simulink model "atrias_2d"  (R2014b)
settings: Solver=ode45  StartTime=0.0  StopTime=t_end
InitFcn:
  | colors
  | simulation_params
  | mechanical_params
StartFcn:
  | tic
StopFcn:
  | stopscript
values from neighbouring files (symbols this model uses):
  A_lpf_velocity = 1 + B1_lpf_velocity + B2_lpf_velocity    [simulation_params.m]
  B1_lpf_velocity = -2*exp(-lpf_damping*fcut_velocity*sample_time)*cos(fcut_velocity*sample_time*sqrt(1-lpf_damping^2))    [simulation_params.m]
  B2_lpf_velocity = exp(-2*lpf_damping*fcut_velocity*sample_time)    [simulation_params.m]
  b_hmotor = 0    [mechanical_params.m]
  b_leg_spring = 0.075*sqrt(k_leg_spring*0.5*.25^2)    [mechanical_params.m]
  b_rotor = 0*60/(2*pi)*9.725e-5    (= 0)    [mechanical_params.m]
  breakaway_friction = [25 25 25 25]    [mechanical_params.m]
  coulomb_friction = [20 20 20 20]    [mechanical_params.m]
  d_com = (d_hip_com_to_torso_com*m_torso)/(m_torso + num_legs*m_hshaft)    [mechanical_params.m]
  delta_phi_max = 160*pi/180    (= 2.79252680319)    [mechanical_params.m]
  delta_phi_min = 25.5*pi/180    (= 0.445058959259)    [mechanical_params.m]
  friction_linear_zone = [0.5 0.5 0.5 0.5].*pi/180    [mechanical_params.m]
  g = 9.81    [mechanical_params.m]
  HIP_MTR_MAX_TORQUE = max_current_hip*Kt_hip*N_h    (= 629.28)    [mechanical_params.m]
  initial_boom_pitch = 0    [mechanical_params.m]
  initial_boom_roll = asin((initial_com_height + boom_mount_to_com + boom_mount_to_center*tan(pitch_mount_angle) - (base_12(2) + yshaft_12(2))) / (l_boom + boom_mount_to_center_diagonal))    [mechanical_params.m]
  initial_boom_yaw = 0    [mechanical_params.m]
  initial_hip_roll = 0*pi/180    (= 0)    [mechanical_params.m]
  initial_winch_angle = -12 * pi/180    (= -0.209439510239)    [mechanical_params.m]
  k_gx = m_total*g/0.01    (= 57082.15332)    [mechanical_params.m]
  k_gy = m_total*g/0.005    (= 114164.30664)    [mechanical_params.m]
  k_leg_spring = 2950    [mechanical_params.m]
  k_phi = 5000    [mechanical_params.m]
  Kb_leg = 0.121    [mechanical_params.m]
  kd_winch = td_winch*kp_winch    (= 989.945961256)    [mechanical_params.m]
  kp_winch = winch_gravity_comp/(3*pi/180)    (= 19798.9192251)    [mechanical_params.m]
  Kt_leg = 0.121    [mechanical_params.m]
  L_leg = 0.102e-3    (= 0.000102)    [mechanical_params.m]
  l_seg = 0.5    [mechanical_params.m]
  LEG_MTR_MAX_TORQUE = max_current_leg * Kt_leg * N    (= 1210)    [mechanical_params.m]
  lowerleg_12 = 0.40    (= 0.4)    [mechanical_params.m]
  m_boom = 4.49    [mechanical_params.m]
  m_fblink = 0.46    [mechanical_params.m]
  m_hshaft = 18    [mechanical_params.m]
  m_lowerleg = 0.4438    [mechanical_params.m]
  m_output_gear = 1e-5    (= 1e-05)    [mechanical_params.m]
  m_rotor = 1e-5    (= 1e-05)    [mechanical_params.m]
  m_shin = 0.75    [mechanical_params.m]
  m_thigh = 0.69    [mechanical_params.m]
  m_torso = 17.5    [mechanical_params.m]
  m_total = num_legs*(m_hshaft + m_thigh + m_lowerleg + m_shin + m_fblink + 2*m_gearing) + m_torso    (= 58.18772)    [mechanical_params.m]
  m_virtual_gear = 1e-5    (= 1e-05)    [mechanical_params.m]
  m_yshaft = 12.89    [mechanical_params.m]
  max_current_leg = 200    [mechanical_params.m]
  max_voltage_leg = 50    [mechanical_params.m]
  mu_hmotor = 0.90    (= 0.9)    [mechanical_params.m]
  mu_motor = 0.85    [mechanical_params.m]
  mu_slide = 0.95    [mechanical_params.m]
  mu_stick = 1.00    (= 1)    [mechanical_params.m]
  N = 50    [mechanical_params.m]
  N_h = r_hip_shaft / r_hip_gearhead    (= 57)    [mechanical_params.m]
  output_sample_time = 1/1000    (= 0.001)    [simulation_params.m]
  phi_max_collision = -5*pi/180    (= -0.0872664625997)    [mechanical_params.m]
  phi_roll_max = pi + 16*pi/180    (= 3.42084533391)    [mechanical_params.m]
  phi_roll_min = pi - 9*pi/180    (= 2.98451302091)    [mechanical_params.m]
  phi_shin_max = 3*pi/2 + 17.5*pi/180    (= 5.01782159948)    [mechanical_params.m]
  phi_shin_min = pi - 45*pi/180    (= 2.35619449019)    [mechanical_params.m]
  phi_thigh_max = pi + 45*pi/180    (= 3.92699081699)    [mechanical_params.m]
  phi_thigh_min = pi/2 - 17.5*pi/180    (= 1.2653637077)    [mechanical_params.m]
  r_hip_gearhead = 0.009525    [mechanical_params.m]
  r_hip_shaft = 0.542925    [mechanical_params.m]
  R_leg = 0.052    [mechanical_params.m]
  r_rotor = 0.001    [mechanical_params.m]
  r_virtual_gear = N*r_rotor    (= 0.05)    [mechanical_params.m]
  s = (x - x1)/(x2 - x1)    [controller.m]
  sample_time = 1/sample_freq    (= 0.001)    [simulation_params.m]
  shin_12 = 0.40    (= 0.4)    [mechanical_params.m]
  shin_initial_l = initial_l_leg_angle + acos(initial_l_leg_length)    [mechanical_params.m]
  shin_initial_r = initial_r_leg_angle + acos(initial_r_leg_length)    [mechanical_params.m]
  thigh_initial_l = initial_l_leg_angle - acos(initial_l_leg_length)    [mechanical_params.m]
  thigh_initial_r = initial_r_leg_angle - acos(initial_r_leg_length)    [mechanical_params.m]
  tile_color = cmap(floor((tile_scale/(max_floor_tile_height+eps))*length(cmap))+1,:)    [mechanical_params.m]
  tile_cross_section = [1.5 0.03; 1.5 0; 3 0; 3 0.03]    [mechanical_params.m]
  tile_delta = [0 1; 0 0; 0 0; 0 1]    [mechanical_params.m]
  tile_scale = zeros(12, 1)    [mechanical_params.m]
  v_gx_max = 0.03    [mechanical_params.m]
  v_gy_max = 0.03    [mechanical_params.m]
  v_phi_max = 1/60    (= 0.0166666666667)    [mechanical_params.m]
  viscous_friction = [0.001 0.001 0.001 0.001]    [mechanical_params.m]
  vLimit = 0.01    [mechanical_params.m]
undefined symbols (not defined in the file or in its folder): base_color_d, boom_color_d, fblink_color_d, floor_color_d, hshaft_color_d, lowerleg_color_d, rad, sgn, shin_color_d, t_friction, thigh_color_d, torso_color_d, X, Y, yshaft_color_d, Z
libraries: sm_lib x196, nesl_utility x125, simulink x48, fl_lib x16, simulink_extras x2, mblibv1 x2, commnoisgen2 x1
(part 5 of 8)

== system atrias_2d/Mechanical Simulation Layer/R Leg/Shin SEA ==
  note: Shin SEA Mechanics
  Shin Gear Torque [Nm] : Inport
  Shin Joint [rad rad/s] : Inport  Port=2
  Demux : Demux  Outputs=2
  Gain : Gain  Gain=k_leg_spring
  Gain1 : Gain  Gain=b_leg_spring
  Initial Gear Angle : Constant  Value=shin_initial_r
  Inverse Gear Ratio2 : Gain  Gain=1/N
  Inverse Gear Ratio3 : Gain  Gain=Kt_leg
  Inverse Gear Ratio4 : Gain  Gain=1/Kt_leg
  Motor Efficiency : Gain  Gain=mu_motor
  Motor Controller : Subsystem  Commented=on
  Motor Electromagnetism : Subsystem  Commented=on
  Rotor Damping : Gain  Gain=b_rotor
  Rotor and Gearing : Subsystem
  Sum : Sum  Inputs=++|
  Sum2 : Sum  Inputs=+|-
  Sum3 : Sum  Inputs=|+-
  Sum4 : Sum  Inputs=+|-
  Sum5 : Sum  Inputs=|++
  Torque Limiter (outside) 2 : Saturate  UpperLimit=LEG_MTR_MAX_TORQUE  LowerLimit=-LEG_MTR_MAX_TORQUE  ZeroCross=off
      settings: AttributesFormatString=Hi: %<UpperLimit>\nLo: %<LowerLimit>
  Rotor Joint Conn : PMIOPort  Port=1  Side=Left
  Shin Joint Torque [Nm] : Outport
  Shin Gear [rad] : Outport  Port=2
  wires:
  Sum2/1 -> Gain/1
  Sum5/1 -> Rotor and Gearing/2(Spring Torque [Nm]), Shin Joint Torque [Nm]/1
  Sum3/1 -> Motor Efficiency/1
  Rotor Damping/1 -> Sum3/2
  Gain/1 -> Sum5/1  "tau_load"
  Gain1/1 -> Sum5/2
  Sum4/1 -> Gain1/1
  Shin Joint [rad rad/s]/1 -> Demux/1
  Demux/1 -> Sum2/2
  Demux/2 -> Sum4/2
  Inverse Gear Ratio3/1 -> Sum3/1
  Initial Gear Angle/1 -> Sum/1
  Sum/1 -> Shin Gear [rad]/1, Sum2/1
  Rotor and Gearing/1(Gearhead Position [rad]) -> Sum/2
  Rotor and Gearing/2(Gearhead Velocity [rad/s]) -> Sum4/1
  Motor Efficiency/1 -> Rotor and Gearing/1(Rotor Torque [Nm])
  Inverse Gear Ratio4/1 -> Inverse Gear Ratio3/1
  Motor Controller/1(Voltage [V]) -> Motor Electromagnetism/1(Voltage [V])
  Motor Electromagnetism/1(Current [A]) -> Motor Controller/2(Measured Current [A])
  Shin Gear Torque [Nm]/1 -> Torque Limiter (outside) 2/1
  Inverse Gear Ratio2/1 -> Inverse Gear Ratio4/1
  Rotor and Gearing/3(Rotor Velocity [rad/s]) -> Rotor Damping/1
  Torque Limiter (outside) 2/1 -> Inverse Gear Ratio2/1
  connections:
  Rotor and Gearing/LConn1 -- Rotor Joint Conn/RConn1

== system atrias_2d/Mechanical Simulation Layer/R Leg/Thigh ==
  CS1 to CS2 : sm_lib/Frames and Transforms/Rigid Transform  TranslationMethod=Cartesian  TranslationLengthUnit=m  TranslationStandardAxis=+Z  TranslationStandardOffset=0  TranslationCartesianOffset=[0 -l_seg 0]  TranslationROffset=0  TranslationROffsetUnits=m  TranslationZOffset=0  TranslationZOffsetUnits=m  TranslationThetaOffset=0  TranslationThetaOffsetUnits=deg  RotationMethod=None  RotationAngleUnits=deg  RotationStandardAxis=+Z  RotationAngle=0  RotationArbitraryAxis=[0 0 1]  FollAlignAxisA=+X  BaseAlignAxisA=+Y  FollAlignAxisB=+Y  BaseAlignAxisB=+Z  RotationMatrix=[1 0 0; 0 1 0; 0 0 1]  BlockFunction=simmechanics.library.frames_transforms.rigid_transform
  Frame Data : Subsystem
  Solid : sm_lib/Body Elements/Solid  InertiaType=Custom  Mass=m_thigh  MassUnits=kg  CenterOfMass=com_thigh  CenterOfMassUnits=m  MomentsOfInertia=i_thigh_moments  MomentsOfInertiaUnits=kg*m^2  ProductsOfInertia=i_thigh_products  ProductsOfInertiaUnits=kg*m^2  DensityBased=on  Density=1000  DensityUnits=kg/(m^3)  GraphicType=FromGeometry  MarkerShape=Sphere  MarkerSize=10  MarkerSizeUnits=m  GraphicVisPropType=AdvancedVisualProperties  GraphicDiffuseColor=thigh_color_d  GraphicSpecularColor=[0.5 0.5 0.5 1.0]  GraphicAmbientColor=[thigh_color_d*0.5 1.0]  GraphicEmissiveColor=[0.0 0.0 0.0 1.0]  GraphicShininess=128  GraphicOpacity=1.0  GeometryShape=FromFile  RectangleSize=[1 1]  RectangleSizeUnits=m  BrickDimensions=[1 1 1]  BrickDimensionUnits=m  CylinderRadius=l_rad  CylinderRadiusUnits=m  CylinderLength=l_seg  CylinderLengthUnits=m  SphereRadius=1  SphereRadiusUnits=m  EllipsoidRadii=[1 1 1]  EllipsoidRadiiUnits=m  ExtrusionCrossSection=[1 1; -1 1; -1 -1; 1 -1]  ExtrusionCrossSectionUnits=m  ExtrusionLength=1  ExtrusionLengthUnits=m  PolygonNumSides=3  PolygonOuterRadius=1  PolygonOuterRadiusUnits=m  ExtGeomFileType=STL  ExtGeomFileName=thigh.stl  ExtGeomFileUnits=m  RevolutionCrossSection=[1 1; 1 -1; 2 -1; 2 1]  RevolutionCrossSectionUnits=m  RevolutionExtent=Full  RevolutionAngle=180  RevolutionAngleUnits=deg  BlockFunction=simmechanics.library.body_elements.solid
  CS1 : PMIOPort  Port=1  Side=Left
  CS2 : PMIOPort  Port=2  Side=Right
  connections:
  CS2/RConn1 -- CS1 to CS2/RConn1
  CS1 to CS2/LConn1 -- Solid/RConn1 -- Frame Data/LConn1 -- CS1/RConn1

== system atrias_2d/Mechanical Simulation Layer/R Leg/Thigh SEA ==
  note: Thigh SEA Mechanics
  Thigh Gear Torque [Nm] : Inport
  Thigh Joint [rad rad/s] : Inport  Port=2
  Continuous Angle : mblibv1/Utilities/Continuous Angle  rad=rad  rads=rad/s
  Demux : Demux  Outputs=2
  Gain : Gain  Gain=k_leg_spring
  Gain1 : Gain  Gain=b_leg_spring
  Initial Gear Angle : Constant  Value=thigh_initial_r
  Inverse Gear Ratio1 : Gain  Gain=1/N
  Inverse Gear Ratio2 : Gain  Gain=Kt_leg
  Inverse Gear Ratio3 : Gain  Gain=1/Kt_leg
  Motor Efficiency : Gain  Gain=mu_motor
  Motor Controller : Subsystem  Commented=on
  Motor Electromagnetism : Subsystem  Commented=on
  Rotor Damping : Gain  Gain=b_rotor
  Rotor and Gearing : Subsystem
  Sum : Sum  Inputs=++|
  Sum2 : Sum  Inputs=+|-
  Sum3 : Sum  Inputs=|+-
  Sum4 : Sum  Inputs=+|-
  Sum5 : Sum  Inputs=|++
  Torque Limiter (outside) 2 : Saturate  UpperLimit=LEG_MTR_MAX_TORQUE  LowerLimit=-LEG_MTR_MAX_TORQUE  ZeroCross=off
      settings: AttributesFormatString=Hi: %<UpperLimit>\nLo: %<LowerLimit>
  Rotor Joint Conn : PMIOPort  Port=1  Side=Left
  Thigh Joint Torque [Nm] : Outport
  Thigh Gear [rad] : Outport  Port=2
  wires:
  Sum2/1 -> Gain/1
  Sum3/1 -> Motor Efficiency/1
  Rotor Damping/1 -> Sum3/2
  Gain/1 -> Sum5/1  "tau_load"
  Gain1/1 -> Sum5/2
  Sum4/1 -> Gain1/1
  Thigh Joint [rad rad/s]/1 -> Demux/1
  Demux/1 -> Sum2/2
  Demux/2 -> Sum4/2
  Inverse Gear Ratio3/1 -> Inverse Gear Ratio2/1
  Inverse Gear Ratio2/1 -> Sum3/1
  Initial Gear Angle/1 -> Sum/1
  Sum/1 -> Thigh Gear [rad]/1, Sum2/1
  Continuous Angle/1 -> Sum/2
  Rotor and Gearing/1(Gearhead Position [rad]) -> Continuous Angle/1
  Motor Controller/1(Voltage [V]) -> Motor Electromagnetism/1(Voltage [V])
  Motor Electromagnetism/1(Current [A]) -> Motor Controller/2(Measured Current [A])
  Thigh Gear Torque [Nm]/1 -> Torque Limiter (outside) 2/1
  Inverse Gear Ratio1/1 -> Inverse Gear Ratio3/1
  Motor Efficiency/1 -> Rotor and Gearing/1(Rotor Torque [Nm])
  Rotor and Gearing/2(Gearhead Velocity [rad/s]) -> Sum4/1, Continuous Angle/2
  Sum5/1 -> Thigh Joint Torque [Nm]/1, Rotor and Gearing/2(Spring Torque [Nm])
  Rotor and Gearing/3(Rotor Velocity [rad/s]) -> Rotor Damping/1
  Torque Limiter (outside) 2/1 -> Inverse Gear Ratio1/1
  connections:
  Rotor and Gearing/LConn1 -- Rotor Joint Conn/RConn1

== system atrias_2d/Mechanical Simulation Layer/Right Hip Roll Joint/Mechanical Limits  ==
  vphi : Inport
  phi : Inport  Port=2
  Compare To Constant5 : simulink/Logic and Bit Operations/Compare To Constant  relop=<=  const=phi_max_collision  OutDataTypeStr=boolean  ZeroCross=off
  Compare To Zero1 : simulink/Logic and Bit Operations/Compare To Zero  relop=<=  OutDataTypeStr=boolean  ZeroCross=off
  Compare To Zero2 : simulink/Logic and Bit Operations/Compare To Zero  relop=<=  OutDataTypeStr=boolean  ZeroCross=off
  Constant1 : Constant  Value=phi_roll_min
  Constant2 : Constant  Value=phi_roll_max
  Enabled Subsystem : Subsystem  TreatAsAtomicUnit=on
  Gain2 : Gain  Gain=-1
  Logical Operator : Logic  Operator=OR  Inputs=1  AllPortsSameDT=off  OutDataTypeStr=boolean
  Mux : Mux  Inputs=2
  Roll Max Collision Model : Subsystem
  Roll Min Collision Model : Subsystem
  Stop Simulation6 : Stop
  Sum1 : Sum  Inputs=-+|
  Sum11 : Sum  Inputs=-|+
  Sum5 : Sum  Inputs=+-|
  tau_reaction : Outport
  wires:
  Sum1/1 -> [col_hip_min], Compare To Zero1/1, Roll Min Collision Model/1(phi [rad])
  Roll Min Collision Model/1(tau_interaction[Nm]) -> Sum11/2
  Compare To Zero1/1 -> Roll Min Collision Model/Enable
  phi/1 -> Sum1/2, Sum5/2
  Logical Operator/1 -> Stop Simulation6/1, Enabled Subsystem/Enable
  [col_hip_max] -> Mux/1
  Mux/1 -> Compare To Constant5/1
  [col_hip_min] -> Mux/2
  Sum11/1 -> tau_reaction/1
  Constant1/1 -> Sum1/1
  Compare To Constant5/1 -> Enabled Subsystem/1(Col_Flags), Logical Operator/1
  Constant2/1 -> Sum5/1
  Sum5/1 -> [col_hip_max], Compare To Zero2/1, Roll Max Collision Model/1(phi [rad])
  Compare To Zero2/1 -> Roll Max Collision Model/Enable
  Roll Max Collision Model/1(tau_interaction[Nm]) -> Sum11/1
  vphi/1 -> Roll Min Collision Model/2(vphi [rad/s]), Gain2/1
  Gain2/1 -> Roll Max Collision Model/2(vphi [rad/s])

== system atrias_2d/Mechanical Simulation Layer/Torso/COM Sensor ==
  Mux : Mux  Inputs=3
  PS-Simulink Converter{1,3..8} (7 alike) : nesl_utility/PS-Simulink Converter  PhysicalDomain=network_engine_domain  SubClassName=ps_output  LeftPortType=input  RightPortType=output  PseudoPeriodic=off  Frequencies=[]  Unit=1  AffineConversion=off
  Transform Sensor : sm_lib/Frames and Transforms/Transform Sensor  MeasurementFrame=World  SenseAngle=off  SenseAxis=off  SenseAngle1=off  SenseAngle2=off  SenseAngle3=off  SenseQ=off  SenseR=off  SenseOmegaX=off  SenseOmegaY=off  SenseOmegaZ=off  SenseOmega1=off  SenseOmega2=off  SenseOmega3=off  SenseQDot=off  SenseRDot=off  SenseAlphaX=off  SenseAlphaY=off  SenseAlphaZ=off  SenseAlpha1=off  SenseAlpha2=off  SenseAlpha3=off  SenseQDDot=off  SenseRDDot=off  SenseX=off  SenseY=on  SenseZ=off  SenseRad=off  SenseAzim=off  SenseDist=off  SenseInc=off  SenseXDot=on  SenseYDot=on  SenseZDot=on  SenseRadDot=off  SenseAzimDot=off  SenseDistDot=off  SenseIncDot=off  SenseXDDot=on  SenseYDDot=on  SenseZDDot=on  SenseRadDDot=off  SenseAzimDDot=off  SenseDistDDot=off  SenseIncDDot=off  BlockFunction=simmechanics.library.frames_transforms.transform_sensor
  Transverse Component : Subsystem
  World Frame : sm_lib/Frames and Transforms/World Frame  BlockFunction=simmechanics.library.frames_transforms.world_frame
  COM : PMIOPort  Port=1  Side=Left
  Acceleration : Outport
  y : Outport  Port=2
  dx : Outport  Port=3
  dy : Outport  Port=4
  wires:
  PS-Simulink Converter5/1 -> Mux/3
  Mux/1 -> Acceleration/1
  PS-Simulink Converter8/1 -> y/1
  PS-Simulink Converter3/1 -> Mux/2
  PS-Simulink Converter4/1 -> Mux/1
  PS-Simulink Converter7/1 -> Transverse Component/1(x)
  Transverse Component/1(transverse) -> dx/1
  [qYaw] -> Transverse Component/3(yaw)
  PS-Simulink Converter1/1 -> dy/1
  PS-Simulink Converter6/1 -> Transverse Component/2(z)
  connections:
  COM/RConn1 -- Transform Sensor/RConn1
  World Frame/RConn1 -- Transform Sensor/LConn1
  PS-Simulink Converter5/LConn1 -- Transform Sensor/RConn8
  PS-Simulink Converter3/LConn1 -- Transform Sensor/RConn7
  PS-Simulink Converter4/LConn1 -- Transform Sensor/RConn6
  PS-Simulink Converter6/LConn1 -- Transform Sensor/RConn5
  PS-Simulink Converter7/LConn1 -- Transform Sensor/RConn3
  PS-Simulink Converter8/LConn1 -- Transform Sensor/RConn2
  PS-Simulink Converter1/LConn1 -- Transform Sensor/RConn4

== system atrias_2d/Mechanical Simulation Layer/Torso/Frame Data ==
  Kinematic Data : ToWorkspace  VariableName=torso_out  SampleTime=output_sample_time
      settings: Save2DSignal=2-D array (concatenate along first dimension)
  Mux : Mux
  PS-Simulink Converter{,1..3} (4 alike) : nesl_utility/PS-Simulink Converter  PhysicalDomain=network_engine_domain  SubClassName=ps_output  LeftPortType=input  RightPortType=output  PseudoPeriodic=off  Frequencies=[]  Unit=1  AffineConversion=off
  Transform Sensor : sm_lib/Frames and Transforms/Transform Sensor  MeasurementFrame=World  SenseAngle=off  SenseAxis=off  SenseAngle1=off  SenseAngle2=off  SenseAngle3=off  SenseQ=on  SenseR=off  SenseOmegaX=off  SenseOmegaY=off  SenseOmegaZ=off  SenseOmega1=off  SenseOmega2=off  SenseOmega3=off  SenseQDot=off  SenseRDot=off  SenseAlphaX=off  SenseAlphaY=off  SenseAlphaZ=off  SenseAlpha1=off  SenseAlpha2=off  SenseAlpha3=off  SenseQDDot=off  SenseRDDot=off  SenseX=on  SenseY=on  SenseZ=on  SenseRad=off  SenseAzim=off  SenseDist=off  SenseInc=off  SenseXDot=off  SenseYDot=off  SenseZDot=off  SenseRadDot=off  SenseAzimDot=off  SenseDistDot=off  SenseIncDot=off  SenseXDDot=off  SenseYDDot=off  SenseZDDot=off  SenseRadDDot=off  SenseAzimDDot=off  SenseDistDDot=off  SenseIncDDot=off  BlockFunction=simmechanics.library.frames_transforms.transform_sensor
  World Frame : sm_lib/Frames and Transforms/World Frame  BlockFunction=simmechanics.library.frames_transforms.world_frame
  Frame : PMIOPort  Port=1  Side=Left
  wires:
  Mux/1 -> Kinematic Data/1
  PS-Simulink Converter/1 -> Mux/1
  PS-Simulink Converter1/1 -> Mux/2
  PS-Simulink Converter2/1 -> Mux/3
  PS-Simulink Converter3/1 -> Mux/4
  connections:
  PS-Simulink Converter3/LConn1 -- Transform Sensor/RConn5
  PS-Simulink Converter2/LConn1 -- Transform Sensor/RConn4
  PS-Simulink Converter1/LConn1 -- Transform Sensor/RConn3
  PS-Simulink Converter/LConn1 -- Transform Sensor/RConn2
  Transform Sensor/RConn1 -- Frame/RConn1
  Transform Sensor/LConn1 -- World Frame/RConn1

== system atrias_2d/Mechanical Simulation Layer/Yaw Shaft/Frame Data ==
  Kinematic Data : ToWorkspace  VariableName=boom_yaw_out  SampleTime=output_sample_time
      settings: Save2DSignal=2-D array (concatenate along first dimension)
  Mux : Mux
  PS-Simulink Converter{,1..3} (4 alike) : nesl_utility/PS-Simulink Converter  PhysicalDomain=network_engine_domain  SubClassName=ps_output  LeftPortType=input  RightPortType=output  PseudoPeriodic=off  Frequencies=[]  Unit=1  AffineConversion=off
  Transform Sensor : sm_lib/Frames and Transforms/Transform Sensor  MeasurementFrame=World  SenseAngle=off  SenseAxis=off  SenseAngle1=off  SenseAngle2=off  SenseAngle3=off  SenseQ=on  SenseR=off  SenseOmegaX=off  SenseOmegaY=off  SenseOmegaZ=off  SenseOmega1=off  SenseOmega2=off  SenseOmega3=off  SenseQDot=off  SenseRDot=off  SenseAlphaX=off  SenseAlphaY=off  SenseAlphaZ=off  SenseAlpha1=off  SenseAlpha2=off  SenseAlpha3=off  SenseQDDot=off  SenseRDDot=off  SenseX=on  SenseY=on  SenseZ=on  SenseRad=off  SenseAzim=off  SenseDist=off  SenseInc=off  SenseXDot=off  SenseYDot=off  SenseZDot=off  SenseRadDot=off  SenseAzimDot=off  SenseDistDot=off  SenseIncDot=off  SenseXDDot=off  SenseYDDot=off  SenseZDDot=off  SenseRadDDot=off  SenseAzimDDot=off  SenseDistDDot=off  SenseIncDDot=off  BlockFunction=simmechanics.library.frames_transforms.transform_sensor
  World Frame : sm_lib/Frames and Transforms/World Frame  BlockFunction=simmechanics.library.frames_transforms.world_frame
  Frame : PMIOPort  Port=1  Side=Left
  wires:
  Mux/1 -> Kinematic Data/1
  PS-Simulink Converter/1 -> Mux/1
  PS-Simulink Converter1/1 -> Mux/2
  PS-Simulink Converter2/1 -> Mux/3
  PS-Simulink Converter3/1 -> Mux/4
  connections:
  PS-Simulink Converter3/LConn1 -- Transform Sensor/RConn5
  PS-Simulink Converter2/LConn1 -- Transform Sensor/RConn4
  PS-Simulink Converter1/LConn1 -- Transform Sensor/RConn3
  PS-Simulink Converter/LConn1 -- Transform Sensor/RConn2
  Transform Sensor/RConn1 -- Frame/RConn1
  Transform Sensor/LConn1 -- World Frame/RConn1

== system atrias_2d/Mechanical Simulation Layer/L Ground Contact/Ground Friction Model/Friction Switch ==
  note: Static/Kinetic Friction Switch
  Slide! : Inport
  Stick! : Inport  Port=2
  Memory : Memory  InheritSampleTime=on
  S-R Flip-Flop : simulink_extras/Flip Flops/S-R Flip-Flop  initial_condition=0
  Terminator : Terminator
  Stiction : Outport
  wires:
  S-R Flip-Flop/1 -> Memory/1
  S-R Flip-Flop/2 -> Terminator/1
  Stick!/1 -> S-R Flip-Flop/1
  Slide!/1 -> S-R Flip-Flop/2
  Memory/1 -> Stiction/1

== system atrias_2d/Mechanical Simulation Layer/L Ground Contact/Ground Friction Model/t-Axis Kinetic Friction Model ==
  note: Kinetic Friction Model
  note: Footpoint Determiner
  note: Sliding Limit Detector
  pos_x [m] : Inport
  vel_x [m/s] : Inport  Port=2
  pos_z [m] : Inport  Port=3
  vel_z [m/s] : Inport  Port=4
  F_Normal [N] : Inport  Port=5
  Enable : EnablePort  StatesWhenEnabling=reset  ZeroCross=off
  Constant : Constant  Value=vLimit
  Constant1 : Constant  Value=eps
  Demux : Demux  Outputs=2
  Divide : Product  Inputs=*/
  FixPt Relational Operator : RelationalOperator  Operator=>  OutDataTypeStr=boolean  ZeroCross=off
  Magnitude : Subsystem
  Memory : Memory  InheritSampleTime=on
  Mux : Mux  Inputs=2
  Negative : simulink/Logic and Bit Operations/Compare To Zero  relop=<  OutDataTypeStr=boolean
  Product : Product  RndMeth=Zero
  Sum : Sum  Inputs=|+-
  Sum1 : Sum  Inputs=|++
  reverse : Gain  Gain=-1
  sliding friction coefficient : Gain  Gain=mu_slide
  posFP_x [m] : Outport  InitialOutput=0
      settings: AttributesFormatString=initial = '%<InitialOutput>'\nwhen disabled = '%<OutputWhenDisabled>'
  posFP_z [m] : Outport  Port=2  InitialOutput=0
      settings: AttributesFormatString=initial = '%<InitialOutput>'\nwhen disabled = '%<OutputWhenDisabled>'
  Stiction! : Outport  Port=3  OutputWhenDisabled=reset  InitialOutput=0
      settings: AttributesFormatString=initial = '%<InitialOutput>'\nwhen disabled = '%<OutputWhenDisabled>'
  Fx_Slide [N] : Outport  Port=4  OutputWhenDisabled=reset  InitialOutput=0
      settings: AttributesFormatString=initial = '%<InitialOutput>'\nwhen disabled = '%<OutputWhenDisabled>'
  Fz_Slide [N] : Outport  Port=5  OutputWhenDisabled=reset  InitialOutput=0
      settings: AttributesFormatString=initial = '%<InitialOutput>'\nwhen disabled = '%<OutputWhenDisabled>'
  wires:
  reverse/1 -> Product/1
  F_Normal [N]/1 -> sliding friction coefficient/1
  pos_x [m]/1 -> posFP_x [m]/1
  sliding friction coefficient/1 -> Product/2
  Divide/1 -> reverse/1
  FixPt Relational Operator/1 -> Stiction!/1
  Memory/1 -> FixPt Relational Operator/2
  Negative/1 -> Memory/1, FixPt Relational Operator/1
  Magnitude/1(Magnitude) -> Sum/1, Sum1/1
  Sum/1 -> Negative/1
  Constant/1 -> Sum/2
  pos_z [m]/1 -> posFP_z [m]/1
  vel_x [m/s]/1 -> Mux/1
  vel_z [m/s]/1 -> Mux/2
  Mux/1 -> Divide/1, Magnitude/1(Vector)
  Constant1/1 -> Sum1/2
  Sum1/1 -> Divide/2
  Product/1 -> Demux/1
  Demux/1 -> Fx_Slide [N]/1
  Demux/2 -> Fz_Slide [N]/1

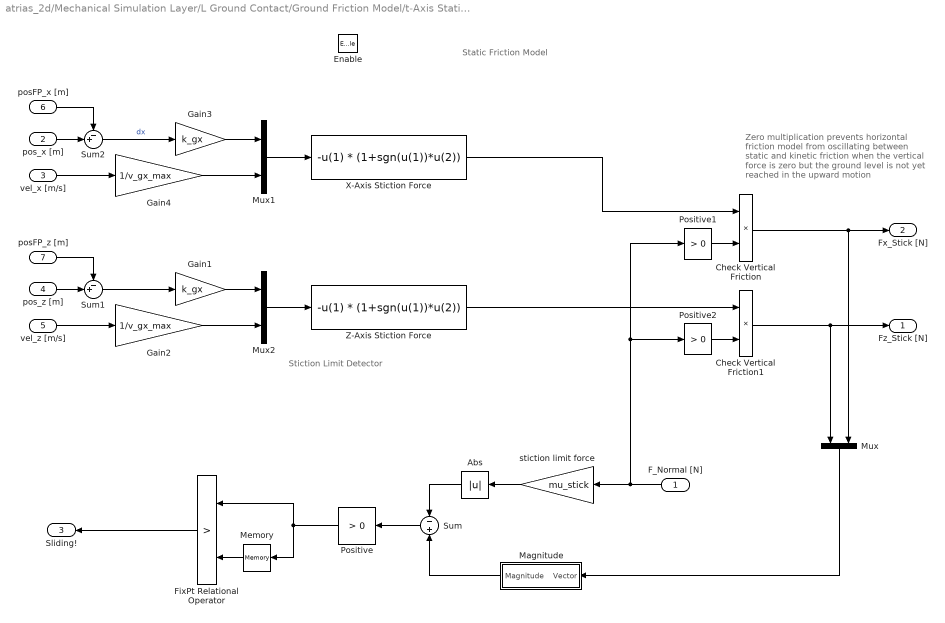
== system atrias_2d/Mechanical Simulation Layer/L Ground Contact/Ground Friction Model/t-Axis Static Friction Model ==
  note: Zero multiplication prevents
      | horizontal friction model from
      | oscillating between static and kinetic
      | friction when the vertical force is zero but
      | the ground level is not yet reached
      | in the upward motion
  note: Stiction Limit Detector
  note: Static Friction Model
  F_Normal [N] : Inport
  pos_x [m] : Inport  Port=2
  vel_x [m/s] : Inport  Port=3
  pos_z [m] : Inport  Port=4
  vel_z [m/s] : Inport  Port=5
  posFP_x [m] : Inport  Port=6
  posFP_z [m] : Inport  Port=7
  Enable : EnablePort  StatesWhenEnabling=reset  ZeroCross=off
  Abs : Abs
  Check Vertical Friction : Product  RndMeth=Zero
  Check Vertical Friction1 : Product  RndMeth=Zero
  FixPt Relational Operator : RelationalOperator  Operator=>  OutDataTypeStr=boolean  ZeroCross=off
  Gain1 : Gain  Gain=k_gx
  Gain2 : Gain  Gain=1/v_gx_max
  Gain3 : Gain  Gain=k_gx
  Gain4 : Gain  Gain=1/v_gx_max
  Magnitude : Subsystem
  Memory : Memory  InheritSampleTime=on
  Mux : Mux  Inputs=2
  Mux1 : Mux  Inputs=2
  Mux2 : Mux  Inputs=2
  Positive : simulink/Logic and Bit Operations/Compare To Zero  relop=>  OutDataTypeStr=boolean
  Positive1 : simulink/Logic and Bit Operations/Compare To Zero  relop=>  OutDataTypeStr=boolean
  Positive2 : simulink/Logic and Bit Operations/Compare To Zero  relop=>  OutDataTypeStr=boolean
  Sum : Sum  Inputs=-+
  Sum1 : Sum  Inputs=-+|
  Sum2 : Sum  Inputs=-+|
  X-Axis Stiction Force : Fcn  Expr=-u(1) * (1+sgn(u(1))*u(2))
  Z-Axis Stiction Force : Fcn  Expr=-u(1) * (1+sgn(u(1))*u(2))
  stiction limit force : Gain  Gain=mu_stick
  Fz_Stick [N] : Outport  OutputWhenDisabled=reset  InitialOutput=0
      settings: AttributesFormatString=when disabled: %<OutputWhenDisabled>\ninitial: %<InitialOutput>
  Fx_Stick [N] : Outport  Port=2  OutputWhenDisabled=reset  InitialOutput=0
      settings: AttributesFormatString=when disabled: %<OutputWhenDisabled>\ninitial: %<InitialOutput>
  Sliding! : Outport  Port=3  OutputWhenDisabled=reset  InitialOutput=0
      settings: AttributesFormatString=when disabled: %<OutputWhenDisabled>\ninitial: %<InitialOutput>
  wires:
  Check Vertical Friction/1 -> Mux/2, Fx_Stick [N]/1
  Positive1/1 -> Check Vertical Friction/2
  X-Axis Stiction Force/1 -> Check Vertical Friction/1
  stiction limit force/1 -> Abs/1
  Abs/1 -> Sum/1
  FixPt Relational Operator/1 -> Sliding!/1
  Gain4/1 -> Mux1/2
  Gain3/1 -> Mux1/1
  Mux1/1 -> X-Axis Stiction Force/1
  Positive/1 -> Memory/1, FixPt Relational Operator/1
  Memory/1 -> FixPt Relational Operator/2
  Sum/1 -> Positive/1
  vel_x [m/s]/1 -> Gain4/1
  posFP_x [m]/1 -> Sum2/1
  pos_x [m]/1 -> Sum2/2
  Sum2/1 -> Gain3/1  "dx"
  F_Normal [N]/1 -> Positive2/1, Positive1/1, stiction limit force/1
  Gain2/1 -> Mux2/2
  Gain1/1 -> Mux2/1
  Mux2/1 -> Z-Axis Stiction Force/1
  vel_z [m/s]/1 -> Gain2/1
  posFP_z [m]/1 -> Sum1/1
  pos_z [m]/1 -> Sum1/2
  Positive2/1 -> Check Vertical Friction1/2
  Z-Axis Stiction Force/1 -> Check Vertical Friction1/1
  Check Vertical Friction1/1 -> Mux/1, Fz_Stick [N]/1
  Magnitude/1(Magnitude) -> Sum/2
  Mux/1 -> Magnitude/1(Vector)
  Sum1/1 -> Gain1/1

== system atrias_2d/Mechanical Simulation Layer/L Leg/Four Bar Link/Frame Data ==
  Kinematic Data : ToWorkspace  VariableName=l_fb_link_out  SampleTime=output_sample_time
      settings: Save2DSignal=2-D array (concatenate along first dimension)
  Mux : Mux
  PS-Simulink Converter{,1..3} (4 alike) : nesl_utility/PS-Simulink Converter  PhysicalDomain=network_engine_domain  SubClassName=ps_output  LeftPortType=input  RightPortType=output  PseudoPeriodic=off  Frequencies=[]  Unit=1  AffineConversion=off
  Transform Sensor : sm_lib/Frames and Transforms/Transform Sensor  MeasurementFrame=World  SenseAngle=off  SenseAxis=off  SenseAngle1=off  SenseAngle2=off  SenseAngle3=off  SenseQ=on  SenseR=off  SenseOmegaX=off  SenseOmegaY=off  SenseOmegaZ=off  SenseOmega1=off  SenseOmega2=off  SenseOmega3=off  SenseQDot=off  SenseRDot=off  SenseAlphaX=off  SenseAlphaY=off  SenseAlphaZ=off  SenseAlpha1=off  SenseAlpha2=off  SenseAlpha3=off  SenseQDDot=off  SenseRDDot=off  SenseX=on  SenseY=on  SenseZ=on  SenseRad=off  SenseAzim=off  SenseDist=off  SenseInc=off  SenseXDot=off  SenseYDot=off  SenseZDot=off  SenseRadDot=off  SenseAzimDot=off  SenseDistDot=off  SenseIncDot=off  SenseXDDot=off  SenseYDDot=off  SenseZDDot=off  SenseRadDDot=off  SenseAzimDDot=off  SenseDistDDot=off  SenseIncDDot=off  BlockFunction=simmechanics.library.frames_transforms.transform_sensor
  World Frame : sm_lib/Frames and Transforms/World Frame  BlockFunction=simmechanics.library.frames_transforms.world_frame
  Frame : PMIOPort  Port=1  Side=Left
  wires:
  Mux/1 -> Kinematic Data/1
  PS-Simulink Converter/1 -> Mux/1
  PS-Simulink Converter1/1 -> Mux/2
  PS-Simulink Converter2/1 -> Mux/3
  PS-Simulink Converter3/1 -> Mux/4
  connections:
  PS-Simulink Converter3/LConn1 -- Transform Sensor/RConn5
  PS-Simulink Converter2/LConn1 -- Transform Sensor/RConn4
  PS-Simulink Converter1/LConn1 -- Transform Sensor/RConn3
  PS-Simulink Converter/LConn1 -- Transform Sensor/RConn2
  Transform Sensor/RConn1 -- Frame/RConn1
  Transform Sensor/LConn1 -- World Frame/RConn1

== system atrias_2d/Mechanical Simulation Layer/L Leg/Lower Leg/Frame Data ==
  Kinematic Data : ToWorkspace  VariableName=l_lower_leg_out  SampleTime=output_sample_time
      settings: Save2DSignal=2-D array (concatenate along first dimension)
  Mux : Mux
  PS-Simulink Converter{,1..3} (4 alike) : nesl_utility/PS-Simulink Converter  PhysicalDomain=network_engine_domain  SubClassName=ps_output  LeftPortType=input  RightPortType=output  PseudoPeriodic=off  Frequencies=[]  Unit=1  AffineConversion=off
  Transform Sensor : sm_lib/Frames and Transforms/Transform Sensor  MeasurementFrame=World  SenseAngle=off  SenseAxis=off  SenseAngle1=off  SenseAngle2=off  SenseAngle3=off  SenseQ=on  SenseR=off  SenseOmegaX=off  SenseOmegaY=off  SenseOmegaZ=off  SenseOmega1=off  SenseOmega2=off  SenseOmega3=off  SenseQDot=off  SenseRDot=off  SenseAlphaX=off  SenseAlphaY=off  SenseAlphaZ=off  SenseAlpha1=off  SenseAlpha2=off  SenseAlpha3=off  SenseQDDot=off  SenseRDDot=off  SenseX=on  SenseY=on  SenseZ=on  SenseRad=off  SenseAzim=off  SenseDist=off  SenseInc=off  SenseXDot=off  SenseYDot=off  SenseZDot=off  SenseRadDot=off  SenseAzimDot=off  SenseDistDot=off  SenseIncDot=off  SenseXDDot=off  SenseYDDot=off  SenseZDDot=off  SenseRadDDot=off  SenseAzimDDot=off  SenseDistDDot=off  SenseIncDDot=off  BlockFunction=simmechanics.library.frames_transforms.transform_sensor
  World Frame : sm_lib/Frames and Transforms/World Frame  BlockFunction=simmechanics.library.frames_transforms.world_frame
  Frame : PMIOPort  Port=1  Side=Left
  wires:
  Mux/1 -> Kinematic Data/1
  PS-Simulink Converter/1 -> Mux/1
  PS-Simulink Converter1/1 -> Mux/2
  PS-Simulink Converter2/1 -> Mux/3
  PS-Simulink Converter3/1 -> Mux/4
  connections:
  PS-Simulink Converter3/LConn1 -- Transform Sensor/RConn5
  PS-Simulink Converter2/LConn1 -- Transform Sensor/RConn4
  PS-Simulink Converter1/LConn1 -- Transform Sensor/RConn3
  PS-Simulink Converter/LConn1 -- Transform Sensor/RConn2
  Transform Sensor/RConn1 -- Frame/RConn1
  Transform Sensor/LConn1 -- World Frame/RConn1

== system atrias_2d/Mechanical Simulation Layer/L Leg/Mechanical Limits/Enabled Subsystem ==
  Col_Flags : Inport
  Enable : EnablePort  StatesWhenEnabling=reset  ZeroCross=off
  To Workspace : ToWorkspace  VariableName=L_collision_flags  SampleTime=-1
  wires:
  Col_Flags/1 -> To Workspace/1

== system atrias_2d/Mechanical Simulation Layer/L Leg/Mechanical Limits/Shin Max Collision Model ==
  note: Mechanical Limits Model
  phi [rad] : Inport
  vphi [rad/s] : Inport  Port=2
  Contact! : EnablePort  StatesWhenEnabling=reset
  Gain3 : Gain  Gain=k_phi
  Gain4 : Gain  Gain=1/v_phi_max
  Mux1 : Mux  Inputs=2
  Reaction Force : Fcn  Expr="- u(1)  *  (1-u(2)) * (u(2)<1)"
  tau_interaction[Nm] : Outport  OutputWhenDisabled=reset  InitialOutput=0
      settings: AttributesFormatString=initial = '%<InitialOutput>'\nwhen disabled = '%<OutputWhenDisabled>'
  wires:
  Gain4/1 -> Mux1/2
  Gain3/1 -> Mux1/1
  Mux1/1 -> Reaction Force/1
  vphi [rad/s]/1 -> Gain4/1
  phi [rad]/1 -> Gain3/1
  Reaction Force/1 -> tau_interaction[Nm]/1

== system atrias_2d/Mechanical Simulation Layer/L Leg/Mechanical Limits/Shin Min Collision Model ==
  note: Mechanical Limits Model
  phi [rad] : Inport
  vphi [rad/s] : Inport  Port=2
  Contact! : EnablePort  StatesWhenEnabling=reset
  Gain3 : Gain  Gain=k_phi
  Gain4 : Gain  Gain=1/v_phi_max
  Mux1 : Mux  Inputs=2
  Reaction Force : Fcn  Expr="- u(1)  *  (1-u(2)) * (u(2)<1)"
  tau_interaction[Nm] : Outport  OutputWhenDisabled=reset  InitialOutput=0
      settings: AttributesFormatString=initial = '%<InitialOutput>'\nwhen disabled = '%<OutputWhenDisabled>'
  wires:
  Gain4/1 -> Mux1/2
  Gain3/1 -> Mux1/1
  Mux1/1 -> Reaction Force/1
  vphi [rad/s]/1 -> Gain4/1
  phi [rad]/1 -> Gain3/1
  Reaction Force/1 -> tau_interaction[Nm]/1

== system atrias_2d/Mechanical Simulation Layer/L Leg/Mechanical Limits/Thigh Max Collision Model ==
  note: Mechanical Limits Model
  phi [rad] : Inport
  vphi [rad/s] : Inport  Port=2
  Contact! : EnablePort  StatesWhenEnabling=reset
  Gain3 : Gain  Gain=k_phi
  Gain4 : Gain  Gain=1/v_phi_max
  Mux1 : Mux  Inputs=2
  Reaction Force : Fcn  Expr="- u(1)  *  (1-u(2)) * (u(2)<1)"
  tau_interaction[Nm] : Outport  OutputWhenDisabled=reset  InitialOutput=0
      settings: AttributesFormatString=initial = '%<InitialOutput>'\nwhen disabled = '%<OutputWhenDisabled>'
  wires:
  Gain4/1 -> Mux1/2
  Gain3/1 -> Mux1/1
  Mux1/1 -> Reaction Force/1
  vphi [rad/s]/1 -> Gain4/1
  phi [rad]/1 -> Gain3/1
  Reaction Force/1 -> tau_interaction[Nm]/1

== system atrias_2d/Mechanical Simulation Layer/L Leg/Mechanical Limits/Thigh Min Collision Model ==
  note: Mechanical Limits Model
  phi [rad] : Inport
  vphi [rad/s] : Inport  Port=2
  Contact! : EnablePort  StatesWhenEnabling=reset
  Gain3 : Gain  Gain=k_phi
  Gain4 : Gain  Gain=1/v_phi_max
  Mux1 : Mux  Inputs=2
  Reaction Force : Fcn  Expr="- u(1)  *  (1-u(2)) * (u(2)<1)"
  tau_interaction[Nm] : Outport  OutputWhenDisabled=reset  InitialOutput=0
      settings: AttributesFormatString=initial = '%<InitialOutput>'\nwhen disabled = '%<OutputWhenDisabled>'
  wires:
  Reaction Force/1 -> tau_interaction[Nm]/1
  phi [rad]/1 -> Gain3/1
  vphi [rad/s]/1 -> Gain4/1
  Mux1/1 -> Reaction Force/1
  Gain3/1 -> Mux1/1
  Gain4/1 -> Mux1/2

== system atrias_2d/Mechanical Simulation Layer/L Leg/Mechanical Limits/Thigh-Shin Collision Model ==
  note: Mechanical Limits Model
  delta_phi [rad] : Inport
  vphi [rad/s] : Inport  Port=2
  Contact! : EnablePort  StatesWhenEnabling=reset
  Gain3 : Gain  Gain=k_phi
  Gain4 : Gain  Gain=1/v_phi_max
  Mux1 : Mux  Inputs=2
  Reaction Force : Fcn  Expr="- u(1)  *  (1-u(2)) * (u(2)<1)"
  tau_interaction[Nm] : Outport  OutputWhenDisabled=reset  InitialOutput=0
      settings: AttributesFormatString=initial = '%<InitialOutput>'\nwhen disabled = '%<OutputWhenDisabled>'
  wires:
  Reaction Force/1 -> tau_interaction[Nm]/1
  delta_phi [rad]/1 -> Gain3/1
  vphi [rad/s]/1 -> Gain4/1
  Mux1/1 -> Reaction Force/1
  Gain3/1 -> Mux1/1
  Gain4/1 -> Mux1/2

== system atrias_2d/Mechanical Simulation Layer/L Leg/Mechanical Limits/Thigh-Shin Collision Model1 ==
  note: Mechanical Limits Model
  delta_phi [rad] : Inport
  vphi [rad/s] : Inport  Port=2
  Contact! : EnablePort  StatesWhenEnabling=reset
  Gain3 : Gain  Gain=k_phi
  Gain4 : Gain  Gain=1/v_phi_max
  Mux1 : Mux  Inputs=2
  Reaction Force : Fcn  Expr="- u(1)  *  (1-u(2)) * (u(2)<1)"
  tau_interaction[Nm] : Outport  OutputWhenDisabled=reset  InitialOutput=0
      settings: AttributesFormatString=initial = '%<InitialOutput>'\nwhen disabled = '%<OutputWhenDisabled>'
  wires:
  Reaction Force/1 -> tau_interaction[Nm]/1
  delta_phi [rad]/1 -> Gain3/1
  vphi [rad/s]/1 -> Gain4/1
  Mux1/1 -> Reaction Force/1
  Gain3/1 -> Mux1/1
  Gain4/1 -> Mux1/2

== system atrias_2d/Mechanical Simulation Layer/L Leg/Shin/Frame Data ==
  Kinematic Data : ToWorkspace  VariableName=l_shin_out  SampleTime=output_sample_time
      settings: Save2DSignal=2-D array (concatenate along first dimension)
  Mux : Mux
  PS-Simulink Converter{,1..3} (4 alike) : nesl_utility/PS-Simulink Converter  PhysicalDomain=network_engine_domain  SubClassName=ps_output  LeftPortType=input  RightPortType=output  PseudoPeriodic=off  Frequencies=[]  Unit=1  AffineConversion=off
  Transform Sensor : sm_lib/Frames and Transforms/Transform Sensor  MeasurementFrame=World  SenseAngle=off  SenseAxis=off  SenseAngle1=off  SenseAngle2=off  SenseAngle3=off  SenseQ=on  SenseR=off  SenseOmegaX=off  SenseOmegaY=off  SenseOmegaZ=off  SenseOmega1=off  SenseOmega2=off  SenseOmega3=off  SenseQDot=off  SenseRDot=off  SenseAlphaX=off  SenseAlphaY=off  SenseAlphaZ=off  SenseAlpha1=off  SenseAlpha2=off  SenseAlpha3=off  SenseQDDot=off  SenseRDDot=off  SenseX=on  SenseY=on  SenseZ=on  SenseRad=off  SenseAzim=off  SenseDist=off  SenseInc=off  SenseXDot=off  SenseYDot=off  SenseZDot=off  SenseRadDot=off  SenseAzimDot=off  SenseDistDot=off  SenseIncDot=off  SenseXDDot=off  SenseYDDot=off  SenseZDDot=off  SenseRadDDot=off  SenseAzimDDot=off  SenseDistDDot=off  SenseIncDDot=off  BlockFunction=simmechanics.library.frames_transforms.transform_sensor
  World Frame : sm_lib/Frames and Transforms/World Frame  BlockFunction=simmechanics.library.frames_transforms.world_frame
  Frame : PMIOPort  Port=1  Side=Left
  wires:
  Mux/1 -> Kinematic Data/1
  PS-Simulink Converter/1 -> Mux/1
  PS-Simulink Converter1/1 -> Mux/2
  PS-Simulink Converter2/1 -> Mux/3
  PS-Simulink Converter3/1 -> Mux/4
  connections:
  PS-Simulink Converter3/LConn1 -- Transform Sensor/RConn5
  PS-Simulink Converter2/LConn1 -- Transform Sensor/RConn4
  PS-Simulink Converter1/LConn1 -- Transform Sensor/RConn3
  PS-Simulink Converter/LConn1 -- Transform Sensor/RConn2
  Transform Sensor/RConn1 -- Frame/RConn1
  Transform Sensor/LConn1 -- World Frame/RConn1

== system atrias_2d/Mechanical Simulation Layer/L Leg/Shin SEA/Motor Controller ==
  Desired Current [A] : Inport
  Measured Current [A] : Inport  Port=2
  Speed [rad/s] : Inport  Port=3
  Ke : Gain  Gain=Kb_leg
  PI Controller : simulink/Continuous/PID Controller  Controller=PI  TimeDomain=Continuous-time  SampleTime=-1  IntegratorMethod=Trapezoidal  FilterMethod=Forward Euler  Form=Parallel  P=0.57  I=0.016  D=0.016  N=10  InitialConditionSource=internal  InitialConditionForIntegrator=0  InitialConditionForFilter=0  ExternalReset=none  ZeroCross=off  LimitOutput=off  UpperSaturationLimit=inf  LowerSaturationLimit=-inf  LinearizeAsGain=on  AntiWindupMode=none  Kb=1  TrackingMode=off  Kt=1  PParamMin=[]  PParamMax=[]  IParamMin=[]  IParamMax=[]  DParamMin=[]  DParamMax=[]  NParamMin=[]  NParamMax=[]  KbParamMin=[]  KbParamMax=[]  KtParamMin=[]  KtParamMax=[]  POutMin=[]  POutMax=[]  IOutMin=[]  IOutMax=[]  DOutMin=[]  DOutMax=[]  NOutMin=[]  NOutMax=[]  KbOutMin=[]  KbOutMax=[]  KtOutMin=[]  KtOutMax=[]  IntegratorOutMin=[]  IntegratorOutMax=[]  FilterOutMin=[]  FilterOutMax=[]  SumOutMin=[]  SumOutMax=[]  SumI1OutMin=[]  SumI1OutMax=[]  SumI2OutMin=[]  SumI2OutMax=[]  SumI3OutMin=[]  SumI3OutMax=[]  SumDOutMin=[]  SumDOutMax=[]  SaturationOutMin=[]  SaturationOutMax=[]  IntegratorContinuousStateAttributes=''  IntegratorStateMustResolveToSignalObject=off  IntegratorRTWStateStorageClass=Auto  FilterContinuousStateAttributes=''  FilterStateMustResolveToSignalObject=off  FilterRTWStateStorageClass=Auto  DifferentiatorICPrevScaledInput=0  DifferentiatorOutMin=[]  DifferentiatorOutMax=[]  UseFilter=on
  Resistance : Gain  Gain=R_leg
  Sum : Sum  Inputs=|+-
  Sum1 : Sum  Inputs=|++
  Sum2 : Sum  Inputs=+|+
  Voltage [V] : Outport
  wires:
  Desired Current [A]/1 -> Sum/1
  Measured Current [A]/1 -> Resistance/1, Sum/2
  Sum/1 -> PI Controller/1
  PI Controller/1 -> Sum1/1
  Speed [rad/s]/1 -> Ke/1
  Sum2/1 -> Sum1/2
  Resistance/1 -> Sum2/1
  Ke/1 -> Sum2/2
  Sum1/1 -> Voltage [V]/1

== system atrias_2d/Mechanical Simulation Layer/L Leg/Shin SEA/Motor Electromagnetism ==
  Voltage [V] : Inport
  Speed [rad/s] : Inport  Port=2
  Add : Sum  Inputs=-+-
  Inductance : Gain  Gain=1/L_leg
  Integrator : Integrator  ZeroCross=off
  Ke : Gain  Gain=Kb_leg
  Resistance : Gain  Gain=R_leg
  Torque Limiter (outside) 1 : Saturate  UpperLimit=max_voltage_leg  LowerLimit=-max_voltage_leg  ZeroCross=off
      settings: AttributesFormatString=Hi: %<UpperLimit>\nLo: %<LowerLimit>
  Torque Limiter (outside) 2 : Saturate  UpperLimit=max_current_leg  LowerLimit=-max_current_leg  ZeroCross=off
      settings: AttributesFormatString=Hi: %<UpperLimit>\nLo: %<LowerLimit>
  Current [A] : Outport
  wires:
  Integrator/1 -> Torque Limiter (outside) 2/1  "I"
  Inductance/1 -> Integrator/1  "d/dt(I)"
  Speed [rad/s]/1 -> Ke/1  "d/dt(theta)"
  Add/1 -> Inductance/1
  Resistance/1 -> Add/1
  Ke/1 -> Add/3
  Voltage [V]/1 -> Torque Limiter (outside) 1/1
  Torque Limiter (outside) 1/1 -> Add/2
  Torque Limiter (outside) 2/1 -> Resistance/1, Current [A]/1
